simulink model "pmsm_with_pwm"  (R2024a)
settings: Solver=ode3  StartTime=0.0  StopTime=10  FixedStep=1e-5  RelTol=1e-3
libraries: spsIGBTDiodeLib x6, simulink x5, spsCurrentMeasurementLib x3, spsAsynchronousMachineSIUnitsLib x1, spsControlledVoltageSourceLib x1, spsPermanentMagnetSynchronousMachineLib x1, sps_lib x1
settings Model: Creator=akpra  LastModifiedBy=akpra

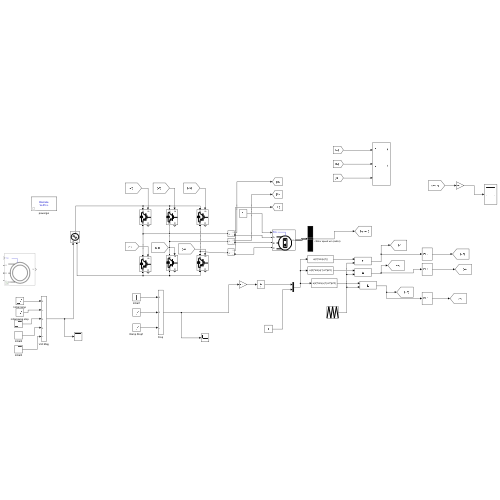
[thumbnail: Simulink's stored preview of the top-level diagram]
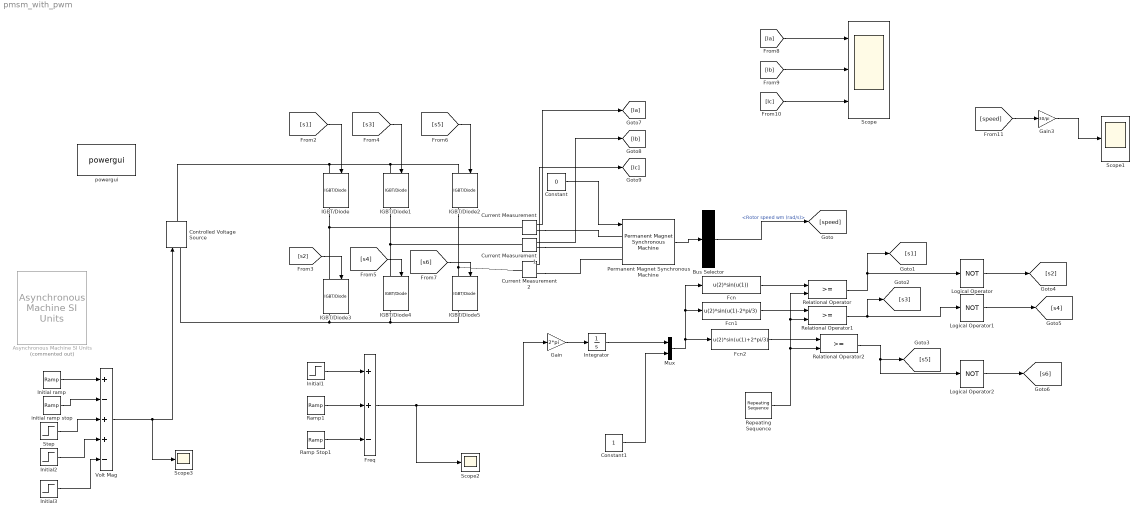
== system pmsm_with_pwm ==
  Asynchronous Machine SI Units : spsAsynchronousMachineSIUnitsLib/Asynchronous Machine SI Units  Commented=on  RotorType=Squirrel-cage  PresetModel=No  MechanicalLoad=Torque Tm  ShowDetailedParameters=on  ReferenceFrame=Rotor  Units=SI  MeasurementBus=off  NominalParameters=[1.845e+04 400 50]  VoltageRatio=1  Stator=[0.5968 0.0003495]  Rotor=[0.6258 0.005473]  Cage1=[0.4155 0.002066]  Cage2=[0.4168 0.0003495]  Lm=0.0354  Mechanical=[0.05 0.005879 2]  PolePairs=2  InitialConditions=[0 0 0 0 0 0 0 0]  SimulateSaturation=off  Saturation=[14.03593122, 27.81365428, 53.79336849, 72.68890987, 97.98006896, 148.6815601, 215.7428561, 302.9841135, 428.7778367 ; 230, 322, 414, 460, 506, 552, 598, 644, 690]  LoadFlowParameters=1492000  TsPowergui=0  TsBlock=-1  IterativeModel=Trapezoidal non iterative  IterativeDiscreteModel=Trapezoidal non iterative  Pmec=1.492e+006
  Bus Selector : BusSelector  OutputSignals=Rotor speed wm (rad/s)
  Constant : Constant  Value=0
  Constant1 : Constant
  Controlled Voltage Source : spsControlledVoltageSourceLib/Controlled Voltage Source  Initialize=on  Source_Type=AC  Amplitude=0  Phase=0  Frequency=0  Measurements=None
  Current Measurement : spsCurrentMeasurementLib/Current Measurement  PhasorSimulation=off  OutputType=Complex  PSBequivalent=0
  Current Measurement1 : spsCurrentMeasurementLib/Current Measurement  PhasorSimulation=off  OutputType=Complex  PSBequivalent=0
  Current Measurement2 : spsCurrentMeasurementLib/Current Measurement  PhasorSimulation=off  OutputType=Complex  PSBequivalent=0
  Fcn : Fcn  Expr=u(2)*sin(u(1))
  Fcn1 : Fcn  Expr=u(2)*sin(u(1)-2*pi/3)
  Fcn2 : Fcn  Expr=u(2)*sin(u(1)+2*pi/3)
  Freq : Sum  Inputs=++-
  Gain : Gain  Gain=2*pi
  Gain3 : Gain  Gain=30/pi
  IGBT/Diode{,1..5} (6 alike) : spsIGBTDiodeLib/IGBT//Diode  Ron=1e-3  Rs=1e5  Cs=inf  Measurements=on
  Initial ramp : simulink/Sources/Ramp  slope=99  start=1  InitialOutput=10
  Initial1 : Step  Time=3  Before=60  After=60  SampleTime=0
  Initial2 : Step  Time=0  Before=10  After=10  SampleTime=0
  Initial3 : Step  Before=10  After=10  SampleTime=0
  Integrator : Integrator
  Logical Operator : Logic  Operator=NOT  AllPortsSameDT=off  OutDataTypeStr=boolean
  Logical Operator1 : Logic  Operator=NOT  AllPortsSameDT=off  OutDataTypeStr=boolean
  Logical Operator2 : Logic  Operator=NOT  AllPortsSameDT=off  OutDataTypeStr=boolean
  Mux : Mux  Inputs=2
  Permanent Magnet Synchronous Machine : spsPermanentMagnetSynchronousMachineLib/Permanent Magnet Synchronous Machine  NbPhases=3  FluxDistribution=Sinusoidal  RotorType=Salient-pole  MechanicalLoad=Torque Tm  PresetModel=No  ShowDetailedParameters=on  MeasurementBus=off  Resistance=1.93  Inductance=8.5e-3  dqInductances=[46.56e-3,79.57e-3]  La=7.3e-3  MachineConstant=Flux linkage established by magnets (V.s)  Flux=0.311  VoltageCst=112.8183  TorqueCst=0.933  Flat=120  Mechanical=[3e-03 1e-3 2 0]  PolePairs=2  InitialConditions=[0,90, 0,0]  InitialConditions5ph=[0 0 0 0 0 0]  RefAngle=Aligned with phase A axis (original Park)  IterativeDiscreteModel=Trapezoidal non iterative  TsBlock=-1  TsPowergui=0
  Ramp Stop1 : simulink/Sources/Ramp  slope=30  start=3  InitialOutput=60
  Ramp1 : simulink/Sources/Ramp  slope=30  start=1  InitialOutput=0
  Relational Operator : RelationalOperator  OutDataTypeStr=boolean  RndMeth=Simplest  InputSameDT=off
  Relational Operator1 : RelationalOperator  OutDataTypeStr=boolean  RndMeth=Simplest  InputSameDT=off
  Relational Operator2 : RelationalOperator  OutDataTypeStr=boolean  RndMeth=Simplest  InputSameDT=off
  Repeating Sequence : simulink/Sources/Repeating Sequence  rep_seq_t=[0 1 2]*(1/5000)  rep_seq_y=[-1 1 -1]
  Scope : Scope  NumInputPorts=3
  Scope1 : Scope
  Scope2 : Scope
  Scope3 : Scope
  Step : Step  Time=3  Before=208  After=208  SampleTime=0
  Volt Mag : Sum  Inputs=+-++-
  initial ramp stop : simulink/Sources/Ramp  slope=99  start=3  InitialOutput=208
  powergui : sps_lib/powergui  Priority=1  SimulationMode=Discrete  SampleTime=1e-5  frequency=60  Iterations=50  frequencyindice=0  Pbase=100e6  ErrMax=1e-4  UnitsV=kV  UnitsW=MW  buscounter=0  FunctionMessages=off  echomessages=off  EnableUseOfTLC=off  CurrentSourceSwitches=off  DisableSnubberDevices=off  DisableRonSwitches=off  DisableVfSwitches=off  DisplayEquations=off  AutomaticDiscreteSolvers=off  SolverType=Tustin  Interpol=off  ExternalGateDelay=off  methode=off  Ts=100  x0status=blocks  SPID=on  SwTol=0  HookPort=off  NonlinearTolerance=1e-4  nMaxIteration=100  ContinueOnMaxIteration=off  RestoreLinks=warning  ResistiveCurrentMeasurement=off  Frange=[0:2:500]  Ylog=off  Xlog=on  ShowGrid=off  save=off  variable=ZData  structure=0  ZoomFFT=off  StartTime=0.0  cycles=1  DisplayStyle=1  fundamental=60  FreqAxis=off  MaxFrequency=1000  frequencyindicesteady=1  RmsSteady=1  display=off
  wires:
  Constant/1 -> Permanent Magnet Synchronous Machine/1
  Permanent Magnet Synchronous Machine/1 -> Bus Selector/1
  Bus Selector/1 -> [speed]  "<Rotor speed wm (rad/s)>"
  Mux/1 -> Fcn1/1, Fcn/1, Fcn2/1
  Fcn/1 -> Relational Operator/1
  Fcn1/1 -> Relational Operator1/1
  Fcn2/1 -> Relational Operator2/1
  Repeating Sequence/1 -> Relational Operator2/2, Relational Operator1/2, Relational Operator/2
  Relational Operator/1 -> [s1], Logical Operator/1
  Relational Operator1/1 -> Logical Operator1/1, [s3]
  Relational Operator2/1 -> Logical Operator2/1, [s5]
  Logical Operator/1 -> [s2]
  Logical Operator1/1 -> [s4]
  Logical Operator2/1 -> [s6]
  [s1] -> IGBT/Diode/1
  [s2] -> IGBT/Diode3/1
  [s3] -> IGBT/Diode1/1
  [s4] -> IGBT/Diode4/1
  [s5] -> IGBT/Diode2/1
  [s6] -> IGBT/Diode5/1
  Current Measurement/1 -> [Ia]
  Current Measurement1/1 -> [Ib]
  Current Measurement2/1 -> [Ic]
  [Ia] -> Scope/1
  [Ib] -> Scope/2
  [Ic] -> Scope/3
  Gain3/1 -> Scope1/1
  [speed] -> Gain3/1
  Initial1/1 -> Freq/1
  Ramp Stop1/1 -> Freq/3
  Ramp1/1 -> Freq/2
  Constant1/1 -> Mux/2
  Gain/1 -> Integrator/1
  Integrator/1 -> Mux/1
  Initial ramp/1 -> Volt Mag/1
  Step/1 -> Volt Mag/3
  Initial2/1 -> Volt Mag/4
  initial ramp stop/1 -> Volt Mag/2
  Volt Mag/1 -> Scope3/1, Controlled Voltage Source/1
  Freq/1 -> Scope2/1, Gain/1
  Initial3/1 -> Volt Mag/5
  connections:
  IGBT/Diode/RConn1 -- Current Measurement/LConn1 -- IGBT/Diode3/LConn1
  IGBT/Diode1/RConn1 -- Current Measurement1/LConn1 -- IGBT/Diode4/LConn1
  IGBT/Diode2/RConn1 -- Current Measurement2/LConn1 -- IGBT/Diode5/LConn1
  IGBT/Diode/LConn1 -- Controlled Voltage Source/RConn1 -- IGBT/Diode2/LConn1 -- IGBT/Diode1/LConn1
  IGBT/Diode3/RConn1 -- Controlled Voltage Source/LConn1 -- IGBT/Diode5/RConn1 -- IGBT/Diode4/RConn1
  Current Measurement/RConn1 -- Permanent Magnet Synchronous Machine/LConn1
  Current Measurement1/RConn1 -- Permanent Magnet Synchronous Machine/LConn2
  Current Measurement2/RConn1 -- Permanent Magnet Synchronous Machine/LConn3
